simulink model "ADC_Model_Three_Phase"  (R2018a)
settings: configuration reference "ModelConfig_var" (kept outside this file)
InitFcn:
  | %% BUS initialization
  | Xabc.A = 0;
  | Xabc.B = 0;
  | Xabc.C = 0;
  | % -------------------------------------------------------------------------
  | Simulink.Bus.createObject(Xabc)
  | XabcBus = slBus1;
  | clear slBus1
model workspace (MAT data in the model file):
  ADCBit_Iabc = 1
  ADCBit_Vdc = 1
  Gain_Iabc = 1
  Gain_Vdc = 1
  Offset_Iabc = 1
  Offset_Vdc = 1
  Out_mode_Iabc = 1
  Out_mode_Vdc = 1
  PGA_Gain_Iabc = 1
  PGA_Gain_Vdc = 1
  Vcc_Iabc = 1
  Vcc_Vdc = 1
settings Model: ParameterArgumentNames=ADCBit_Iabc,ADCBit_Vdc,Gain_Iabc,Gain_Vdc,Offset_Iabc,Offset_Vdc,Out_mode_Iabc,Out_mode_Vdc,PGA_Gain_Iabc,PGA_Gain_Vdc,Vcc_Iabc,Vcc_Vdc  OrderedModelArguments=off  Creator=BEDNASA  LastModifiedBy=BEDNASA
settings ConfigSetRef: SourceLocation=Base Workspace

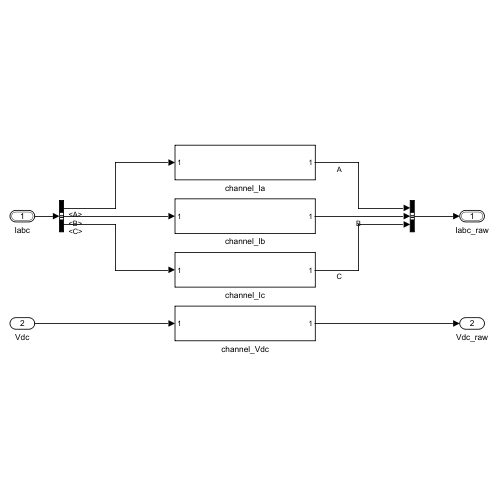
[thumbnail: Simulink's stored preview of the top-level diagram]
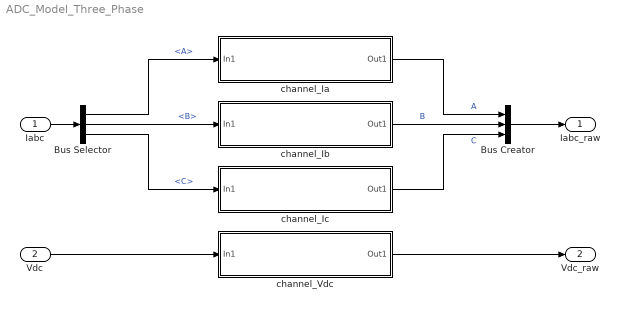
== system ADC_Model_Three_Phase ==
  Iabc : Inport  OutDataTypeStr=Bus: XabcBus
  Vdc : Inport  Port=2
  Bus Creator : BusCreator  Inputs=3  OutDataTypeStr=Bus: XabcBus
  Bus Selector : BusSelector  OutputSignals=A,B,C
  channel_Ia : Subsystem  mask(ADC model){Out_Mode=Out_mode_Iabc, Gain=Gain_Iabc, Offset=Offset_Iabc, Vcc=Vcc_Iabc, ADCBit=ADCBit_Iabc, PGA_Gain=PGA_Gain_Iabc}
      mask prompts: Out_Mode "Output Mode"
      mask help: Atomic ADC model utlized in custom blocks for single and three phase drive systems
      mask TypeOptions Out_Mode: MATLAB Function/Out_Mode
      mask TypeOptions Gain: MATLAB Function/Gain
      mask TypeOptions Offset: MATLAB Function/Offset
      mask TypeOptions Vcc: MATLAB Function/Vcc
      mask TypeOptions ADCBit: MATLAB Function/ADCBit
      mask TypeOptions PGA_Gain: MATLAB Function/PGA_Gain
      mask DialogControl Container3 Prompt: SIL (0) \ RT PIL (1)
  channel_Ib : Subsystem  mask(ADC model){Out_Mode=Out_mode_Iabc, Gain=Gain_Iabc, Offset=Offset_Iabc, Vcc=Vcc_Iabc, ADCBit=ADCBit_Iabc, PGA_Gain=PGA_Gain_Iabc}
      mask prompts: Out_Mode "Output Mode"
      mask help: Atomic ADC model utlized in custom blocks for single and three phase drive systems
      mask TypeOptions Out_Mode: MATLAB Function/Out_Mode
      mask TypeOptions Gain: MATLAB Function/Gain
      mask TypeOptions Offset: MATLAB Function/Offset
      mask TypeOptions Vcc: MATLAB Function/Vcc
      mask TypeOptions ADCBit: MATLAB Function/ADCBit
      mask TypeOptions PGA_Gain: MATLAB Function/PGA_Gain
      mask DialogControl Container3 Prompt: SIL (0) \ RT PIL (1)
  channel_Ic : Subsystem  mask(ADC model){Out_Mode=Out_mode_Iabc, Gain=Gain_Iabc, Offset=Offset_Iabc, Vcc=Vcc_Iabc, ADCBit=ADCBit_Iabc, PGA_Gain=PGA_Gain_Iabc}
      mask prompts: Out_Mode "Output Mode"
      mask help: Atomic ADC model utlized in custom blocks for single and three phase drive systems
      mask TypeOptions Out_Mode: MATLAB Function/Out_Mode
      mask TypeOptions Gain: MATLAB Function/Gain
      mask TypeOptions Offset: MATLAB Function/Offset
      mask TypeOptions Vcc: MATLAB Function/Vcc
      mask TypeOptions ADCBit: MATLAB Function/ADCBit
      mask TypeOptions PGA_Gain: MATLAB Function/PGA_Gain
      mask DialogControl Container3 Prompt: SIL (0) \ RT PIL (1)
  channel_Vdc : Subsystem  mask(ADC model){Out_Mode=Out_mode_Vdc, Gain=Gain_Vdc, Offset=Offset_Vdc, Vcc=Vcc_Vdc, ADCBit=ADCBit_Vdc, PGA_Gain=PGA_Gain_Vdc}
      mask prompts: Out_Mode "Output Mode"
      mask help: Atomic ADC model utlized in custom blocks for single and three phase drive systems
      mask TypeOptions Out_Mode: MATLAB Function/Out_Mode
      mask TypeOptions Gain: MATLAB Function/Gain
      mask TypeOptions Offset: MATLAB Function/Offset
      mask TypeOptions Vcc: MATLAB Function/Vcc
      mask TypeOptions ADCBit: MATLAB Function/ADCBit
      mask TypeOptions PGA_Gain: MATLAB Function/PGA_Gain
      mask DialogControl Container3 Prompt: SIL (0) \ RT PIL (1)
  Iabc_raw : Outport  OutDataTypeStr=Bus: XabcBus
  Vdc_raw : Outport  Port=2
  wires:
  channel_Ib/1(Out1) -> Bus Creator/2  "B"
  Bus Creator/1 -> Iabc_raw/1
  Vdc/1 -> channel_Vdc/1(In1)
  channel_Ia/1(Out1) -> Bus Creator/1  "A"
  Bus Selector/2 -> channel_Ib/1(In1)  "<B>"
  channel_Vdc/1(Out1) -> Vdc_raw/1
  Bus Selector/1 -> channel_Ia/1(In1)  "<A>"
  Bus Selector/3 -> channel_Ic/1(In1)  "<C>"
  Iabc/1 -> Bus Selector/1
  channel_Ic/1(Out1) -> Bus Creator/3  "C"

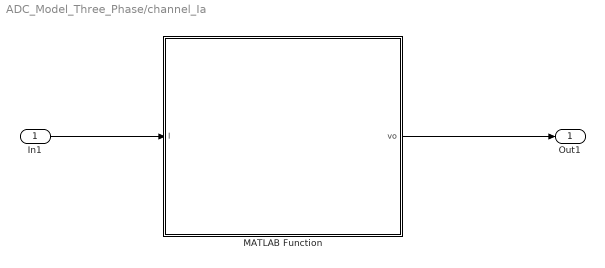
== system ADC_Model_Three_Phase/channel_Ia ==
  In1 : Inport
  MATLAB Function : MATLAB Function  TreatAsAtomicUnit=on  mask(ADC model){Out_Mode=Out_Mode, Gain=Gain, Offset=Offset, Vcc=Vcc, ADCBit=ADCBit, PGA_Gain=PGA_Gain}
      mask prompts: Out_Mode "Output Mode"
      mask help: Atomic ADC model utlized in custom blocks for single and three phase drive systems
  Out1 : Outport
  wires:
  In1/1 -> MATLAB Function/1(I)
  MATLAB Function/1(vo) -> Out1/1

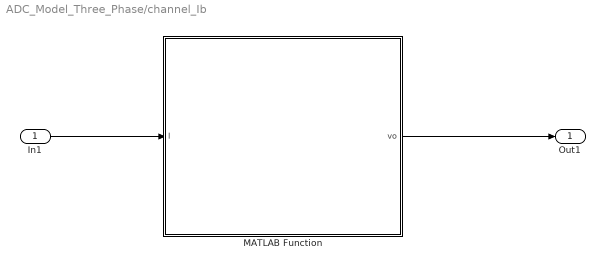
== system ADC_Model_Three_Phase/channel_Ib ==
  In1 : Inport
  MATLAB Function : MATLAB Function  TreatAsAtomicUnit=on  mask(ADC model){Out_Mode=Out_Mode, Gain=Gain, Offset=Offset, Vcc=Vcc, ADCBit=ADCBit, PGA_Gain=PGA_Gain}
      mask prompts: Out_Mode "Output Mode"
      mask help: Atomic ADC model utlized in custom blocks for single and three phase drive systems
  Out1 : Outport
  wires:
  In1/1 -> MATLAB Function/1(I)
  MATLAB Function/1(vo) -> Out1/1

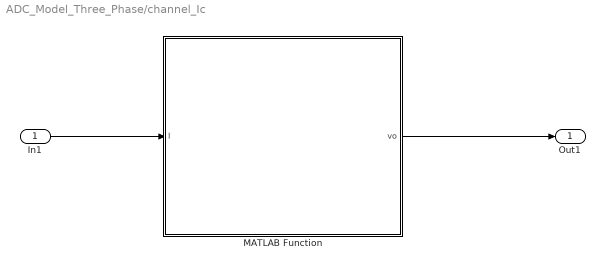
== system ADC_Model_Three_Phase/channel_Ic ==
  In1 : Inport
  MATLAB Function : MATLAB Function  TreatAsAtomicUnit=on  mask(ADC model){Out_Mode=Out_Mode, Gain=Gain, Offset=Offset, Vcc=Vcc, ADCBit=ADCBit, PGA_Gain=PGA_Gain}
      mask prompts: Out_Mode "Output Mode"
      mask help: Atomic ADC model utlized in custom blocks for single and three phase drive systems
  Out1 : Outport
  wires:
  In1/1 -> MATLAB Function/1(I)
  MATLAB Function/1(vo) -> Out1/1

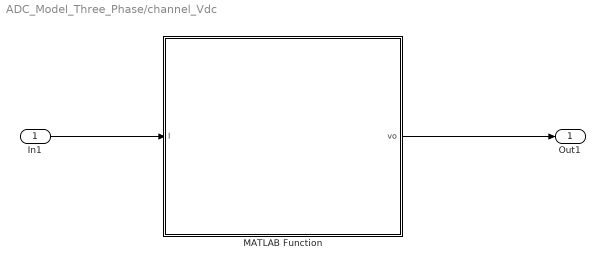
== system ADC_Model_Three_Phase/channel_Vdc ==
  In1 : Inport
  MATLAB Function : MATLAB Function  TreatAsAtomicUnit=on  mask(ADC model){Out_Mode=Out_Mode, Gain=Gain, Offset=Offset, Vcc=Vcc, ADCBit=ADCBit, PGA_Gain=PGA_Gain}
      mask prompts: Out_Mode "Output Mode"
      mask help: Atomic ADC model utlized in custom blocks for single and three phase drive systems
  Out1 : Outport
  wires:
  In1/1 -> MATLAB Function/1(I)
  MATLAB Function/1(vo) -> Out1/1

== matlab function ADC_Model_Three_Phase/channel_Ia/MATLAB Function ==
  data: I input; vo output; Gain parameter; Offset parameter; Vcc parameter; ADCBit parameter; PGA_Gain parameter; Out_Mode parameter
function vo = GetADCRawData(I, Gain, Offset, Vcc, ADCBit, PGA_Gain, Out_Mode)

%Vcc = 1;
%out_mode = 0;
%ADCBit = 12;


%Vout = C1*I+C2;
%Vout_PIL = 1;

Vout=Gain * I + Offset;
Vout_PIL = (Gain/PGA_Gain) * I + Offset/PGA_Gain;

if (Vout > Vcc)
    Vout = Vcc;
elseif (Vout < 0)
    Vout = 0;
end

if Out_Mode == 0        % ADC_counts
    vo = round((Vout/Vcc) * (2^ADCBit));
elseif Out_Mode == 1    % ADC_voltage
    vo = Vout_PIL;
else 
    vo = 0;
end


% function AD_count  = GetADCRawData(in_analog, Gain, Offset, Vcc, ADCbit)
% %% Sensor model with ADC
% % Sensor voltage equation V_out = Gain * in_analog + Offset
% 
% V_out = Gain * in_analog + Offset;
% 
% if (V_out > Vcc)
%     V_out = Vcc;
% elseif (V_out < 0)
%     V_out = 0;
% end
% 
% %% AD Counts
% AD_count = round((V_out/Vcc) * (2^ADCbit));
% end

== matlab function ADC_Model_Three_Phase/channel_Vdc/MATLAB Function ==
  data: I input; vo output; Gain parameter; Offset parameter; Vcc parameter; ADCBit parameter; PGA_Gain parameter; Out_Mode parameter
function vo = GetADCRawData(I, Gain, Offset, Vcc, ADCBit, PGA_Gain, Out_Mode)

%Vcc = 1;
%out_mode = 0;
%ADCBit = 12;


%Vout = C1*I+C2;
%Vout_PIL = 1;

Vout=Gain * I + Offset;
Vout_PIL = (Gain/PGA_Gain) * I + Offset/PGA_Gain;

if (Vout > Vcc)
    Vout = Vcc;
elseif (Vout < 0)
    Vout = 0;
end

if Out_Mode == 0        % ADC_counts
    vo = round((Vout/Vcc) * (2^ADCBit));
elseif Out_Mode == 1    % ADC_voltage
    vo = Vout_PIL;
else 
    vo = 0;
end


% function AD_count  = GetADCRawData(in_analog, Gain, Offset, Vcc, ADCbit)
% %% Sensor model with ADC
% % Sensor voltage equation V_out = Gain * in_analog + Offset
% 
% V_out = Gain * in_analog + Offset;
% 
% if (V_out > Vcc)
%     V_out = Vcc;
% elseif (V_out < 0)
%     V_out = 0;
% end
% 
% %% AD Counts
% AD_count = round((V_out/Vcc) * (2^ADCbit));
% end

== matlab function ADC_Model_Three_Phase/channel_Ib/MATLAB Function ==
  data: I input; vo output; Gain parameter; Offset parameter; Vcc parameter; ADCBit parameter; PGA_Gain parameter; Out_Mode parameter
function vo = GetADCRawData(I, Gain, Offset, Vcc, ADCBit, PGA_Gain, Out_Mode)

%Vcc = 1;
%out_mode = 0;
%ADCBit = 12;


%Vout = C1*I+C2;
%Vout_PIL = 1;

Vout=Gain * I + Offset;
Vout_PIL = (Gain/PGA_Gain) * I + Offset/PGA_Gain;

if (Vout > Vcc)
    Vout = Vcc;
elseif (Vout < 0)
    Vout = 0;
end

if Out_Mode == 0        % ADC_counts
    vo = round((Vout/Vcc) * (2^ADCBit));
elseif Out_Mode == 1    % ADC_voltage
    vo = Vout_PIL;
else 
    vo = 0;
end


% function AD_count  = GetADCRawData(in_analog, Gain, Offset, Vcc, ADCbit)
% %% Sensor model with ADC
% % Sensor voltage equation V_out = Gain * in_analog + Offset
% 
% V_out = Gain * in_analog + Offset;
% 
% if (V_out > Vcc)
%     V_out = Vcc;
% elseif (V_out < 0)
%     V_out = 0;
% end
% 
% %% AD Counts
% AD_count = round((V_out/Vcc) * (2^ADCbit));
% end

== matlab function ADC_Model_Three_Phase/channel_Ic/MATLAB Function ==
  data: I input; vo output; Gain parameter; Offset parameter; Vcc parameter; ADCBit parameter; PGA_Gain parameter; Out_Mode parameter
function vo = GetADCRawData(I, Gain, Offset, Vcc, ADCBit, PGA_Gain, Out_Mode)

%Vcc = 1;
%out_mode = 0;
%ADCBit = 12;


%Vout = C1*I+C2;
%Vout_PIL = 1;

Vout=Gain * I + Offset;
Vout_PIL = (Gain/PGA_Gain) * I + Offset/PGA_Gain;

if (Vout > Vcc)
    Vout = Vcc;
elseif (Vout < 0)
    Vout = 0;
end

if Out_Mode == 0        % ADC_counts
    vo = round((Vout/Vcc) * (2^ADCBit));
elseif Out_Mode == 1    % ADC_voltage
    vo = Vout_PIL;
else 
    vo = 0;
end


% function AD_count  = GetADCRawData(in_analog, Gain, Offset, Vcc, ADCbit)
% %% Sensor model with ADC
% % Sensor voltage equation V_out = Gain * in_analog + Offset
% 
% V_out = Gain * in_analog + Offset;
% 
% if (V_out > Vcc)
%     V_out = Vcc;
% elseif (V_out < 0)
%     V_out = 0;
% end
% 
% %% AD Counts
% AD_count = round((V_out/Vcc) * (2^ADCbit));
% end
